simulink model "Push_Button_mode"  (R2015b)
settings: Solver=FixedStepDiscrete  StartTime=0.0  StopTime=10.0  RelTol=1e-3
libraries: stm32f4lib x3
settings Model: Creator=ronak  LastModifiedBy=ronak
settings OptimizationCC: OptimizeModelRefInitCode=on  LifeSpan=1  MaxStackSize=64
settings HardwareCC: ProdBitPerPointer=32  ProdLargestAtomicInteger=Long  ProdLargestAtomicFloat=Double  ProdWordSize=32  ProdHWDeviceType=ARM Compatible->ARM Cortex
settings RTWCC: SystemTargetFile=ert.tlc  TemplateMakefile=ert_default_tmf  Description=Embedded Coder  Toolchain=GNU Tools for ARM Embedded Processors
settings CodeAppCC: IgnoreCustomStorageClasses=off
settings ERTTargetCC: GenerateSampleERTMain=on

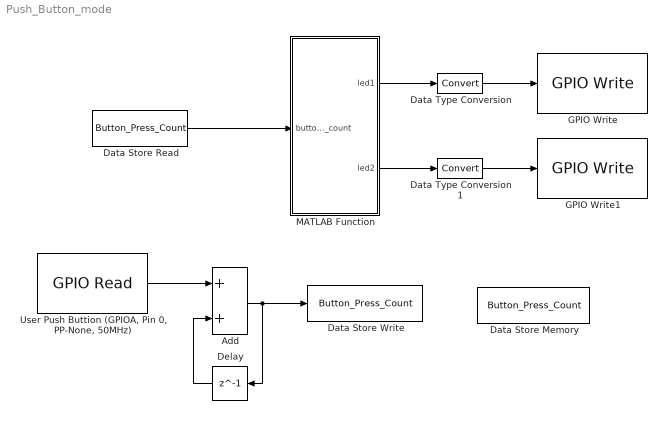
== system Push_Button_mode ==
  Add : Sum
  Data Store Memory : DataStoreMemory  DataStoreName=Button_Press_Count  ReadBeforeWriteMsg=warning  WriteAfterWriteMsg=warning  WriteAfterReadMsg=warning  OutDataTypeStr=uint8
      settings: RTWStateStorageClass=ExportedGlobal
  Data Store Read : DataStoreRead  DataStoreName=Button_Press_Count
  Data Store Write : DataStoreWrite  DataStoreName=Button_Press_Count
  Data Type Conversion : DataTypeConversion
  Data Type Conversion1 : DataTypeConversion
  Delay : Delay  DelayLength=1  InitialCondition=0
  GPIO Write : stm32f4lib/GPIO Write  gpio_name=GPIOD  pin_number=12  pupd_reg=0  otype_reg=0  ospeed_reg=0  gpio_init_out=off  toggle_pin=off
  GPIO Write1 : stm32f4lib/GPIO Write  gpio_name=GPIOD  pin_number=13  pupd_reg=0  otype_reg=0  ospeed_reg=0  gpio_init_out=off  toggle_pin=off
  MATLAB Function : MATLAB Function  TreatAsAtomicUnit=on
  "User Push Buttion (GPIOA, Pin 0, PP-None, 50MHz)" : stm32f4lib/GPIO Read  gpio_name=GPIOA  pin_number=0  sample_time=0.1  pupd_reg=0  otype_reg=0  ospeed_reg=0
  wires:
  "User Push Buttion (GPIOA, Pin 0, PP-None, 50MHz)"/1 -> Add/1
  Add/1 -> Delay/1, Data Store Write/1
  Data Store Read/1 -> MATLAB Function/1(button_count)
  MATLAB Function/1(led1) -> Data Type Conversion/1
  MATLAB Function/2(led2) -> Data Type Conversion1/1
  Data Type Conversion/1 -> GPIO Write/1
  Data Type Conversion1/1 -> GPIO Write1/1
  Delay/1 -> Add/2

== matlab function Push_Button_mode/MATLAB Function ==
  data: button_count input; led1 output; led2 output
function [led1, led2] = fcn(button_count)
%#codegen
mod_button = mod(button_count,4);

switch mod_button
    case 0
        led1 = 0;
        led2 = 0;
    case 1
        led1 = 0;
        led2 = 1;
    case 2
        led1 = 1;
        led2 = 0;
    case 3
        led1 = 1;
        led2 = 1;
    otherwise
        led1 = 0;
        led2 = 0;
end
end
